simulink model "SWC_APP_type"  (R2024a)
settings: Solver=FixedStepDiscrete  StartTime=0.0  StopTime=10.0  FixedStep=0.001  RelTol=1e-3
values from neighbouring files (symbols this model uses):
  TRUE = boolean( 1 )    [vcu_local_hdr.m]
undefined symbols (not defined in the file or in its folder): KAPP_ADCKL15_enum, KAPP_ADCKL30_enum, KFOC_ADCFlyBackTemp_enum, KFOC_ADCMCUTemp_enum, KFOC_ADCMotorUTemp_enum, KFOC_ADCMotorVTemp_enum, KFOC_ADCMotorWTemp_enum, KFOC_ADCOilTemp_enum, KFOC_ADCSicUTemp_enum, KFOC_ADCSicVTemp_enum, KFOC_ADCSicWTemp_enum, KOPM_FakeKL15_flg
libraries: FVT_lib x19, crm_grc x1, eop_grc x1, halin x1, halout x1, inp x1, llc_grc x1, opm_grc x1, syl_grc x1, dgl_grc x1
(part 1 of 2)
settings Model: DataDictionary=APPTypes.sldd  Creator=FVT22063  LastModifiedBy=FVT24180
settings DataIOCC: SaveFormat=StructureWithTime
settings OptimizationCC: DefaultParameterBehavior=Inlined  EnhancedBackFolding=on  PassReuseOutputArgsAs=Individual arguments  ZeroExternalMemoryAtStartup=off  ZeroInternalMemoryAtStartup=off  OptimizeBlockOrder=speed  DifferentSizesBufferReuse=on  OptimizationCustomize=off  EfficientTunableParamExpr=on
settings DebuggingCC: ParameterTunabilityLossMsg=error
settings HardwareCC: ProdBitPerPointer=32  ProdBitPerSizeT=32  ProdBitPerPtrDiffT=32  ProdLargestAtomicInteger=Long  ProdLargestAtomicFloat=Double  ProdWordSize=32  ProdLongLongMode=on  ProdHWDeviceType=ARM Compatible->ARM Cortex-M
settings ModelReferenceCC: ModelReferenceNumInstancesAllowed=Single
settings SFSimCC: SimCustomHeaderCode="#include \"FVTMC_API.h\""  SimUserSources=FVTMC_API.c  MATLABDynamicMemAlloc=off
settings RTWCC: Description=AUTOSAR  SystemTargetFile=autosar.tlc  GenCodeOnly=on  TemplateMakefile=ert_default_tmf  PortableWordSizes=on
settings CodeAppCC: ForceParamTrailComments=on  IgnoreCustomStorageClasses=off  OperatorAnnotations=on  SimulinkDataObjDesc=on  SFDataObjDesc=on  InsertBlockDesc=on
settings STFCustomTargetCC: UtilityFuncGeneration=Shared location  MultiwordLength=256  ParMdlRefBuildCompliant=on  CompOptLevelCompliant=on  IncludeMdlTerminateFcn=off  CombineOutputUpdateFcns=on  SuppressErrorStatus=on  ERTCustomFileBanners=on  SupportNonFinite=off  SupportComplex=off  SupportContinuousTime=off  SupportNonInlinedSFcns=off  RemoveResetFunc=on  MATLABClassNameForMDSCustomization=Simulink.SoftwareTarget.ERTCustomization  AutosarCompliant=on  GRTInterface=off  GenerateSharedConstants=off  LookupTableObjectStructAxisOrder=2,1,3,4,...  LUTObjectStructOrderEvenSpacing=Size,Table,Breakpoints  SystemTargetFile=autosar.tlc
settings ERTTargetCC: TargetLangStandard=C99 (ISO)  UtilityFuncGeneration=Shared location  ConcurrentExecutionCompliant=off  IncludeMdlTerminateFcn=off  SuppressErrorStatus=on  SupportNonFinite=off  SupportComplex=off  ModelStepFunctionPrototypeControlCompliant=off  CPPClassGenCompliant=off  AutosarCompliant=on  GenerateSharedConstants=off  LookupTableObjectStructAxisOrder=2,1,3,4,...  LUTObjectStructOrderEvenSpacing=Size,Table,Breakpoints  GenerateASAP2=on  InlinedParameterPlacement=NonHierarchical  ERTCustomFileTemplate=example_file_process.tlc  ConvertIfToSwitch=off  SuppressUnreachableDefaultCases=off  BooleanTrueId=true_MatlabRTW  BooleanFalseId=false_MatlabRTW

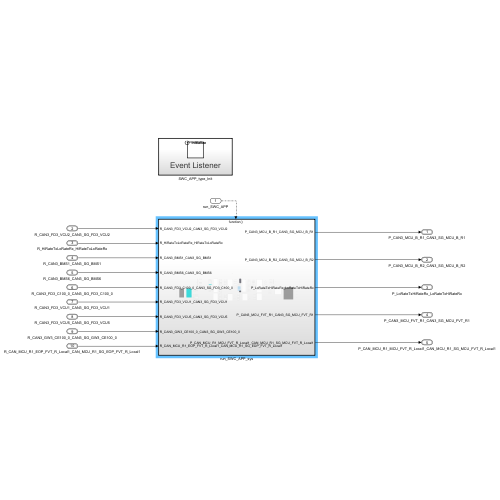
[thumbnail: Simulink's stored preview of the top-level diagram]
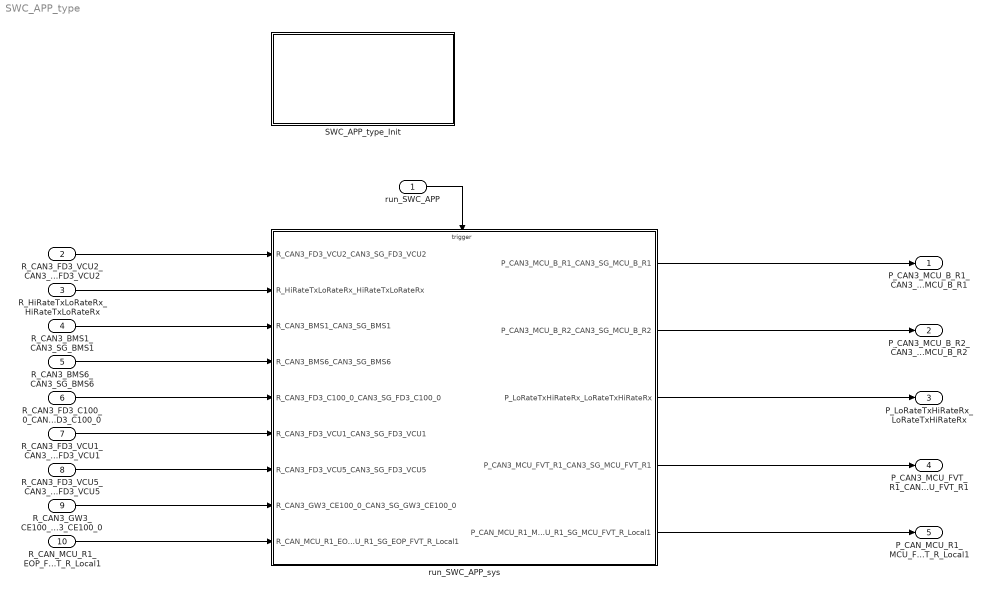
== system SWC_APP_type ==
  run_SWC_APP : Inport  SampleTime=0.001  OutputFunctionCall=on
  R_CAN3_FD3_VCU2_CAN3_SG_FD3_VCU2 : Inport  Port=2  OutDataTypeStr=Bus: DT_CAN3_SG_FD3_VCU2  PortDimensions=1  BusOutputAsStruct=on
  R_HiRateTxLoRateRx_HiRateTxLoRateRx : Inport  Port=3  OutDataTypeStr=Bus: DT_HiRateTxLoRateRx  PortDimensions=1  BusOutputAsStruct=on
  R_CAN3_BMS1_CAN3_SG_BMS1 : Inport  Port=4  OutDataTypeStr=Bus: DT_CAN3_SG_BMS1  PortDimensions=1  BusOutputAsStruct=on
  R_CAN3_BMS6_CAN3_SG_BMS6 : Inport  Port=5  OutDataTypeStr=Bus: DT_CAN3_SG_BMS6  PortDimensions=1  BusOutputAsStruct=on
  R_CAN3_FD3_C100_0_CAN3_SG_FD3_C100_0 : Inport  Port=6  OutDataTypeStr=Bus: DT_CAN3_SG_FD3_C100_0  PortDimensions=1  BusOutputAsStruct=on
  R_CAN3_FD3_VCU1_CAN3_SG_FD3_VCU1 : Inport  Port=7  OutDataTypeStr=Bus: DT_CAN3_SG_FD3_VCU1  PortDimensions=1  BusOutputAsStruct=on
  R_CAN3_FD3_VCU5_CAN3_SG_FD3_VCU5 : Inport  Port=8  OutDataTypeStr=Bus: DT_CAN3_SG_FD3_VCU5  PortDimensions=1  BusOutputAsStruct=on
  R_CAN3_GW3_CE100_0_CAN3_SG_GW3_CE100_0 : Inport  Port=9  OutDataTypeStr=Bus: DT_CAN3_SG_GW3_CE100_0  PortDimensions=1  BusOutputAsStruct=on
  R_CAN_MCU_R1_EOP_FVT_R_Local1_CAN_MCU_R1_SG_EOP_FVT_R_Local1 : Inport  Port=10  OutDataTypeStr=Bus: DT_CAN_MCU_R1_SG_EOP_FVT_R_Local1  PortDimensions=1  BusOutputAsStruct=on
  SWC_APP_type_Init : Subsystem
  run_SWC_APP_sys : Subsystem
  P_CAN3_MCU_B_R1_CAN3_SG_MCU_B_R1 : Outport  OutDataTypeStr=Bus: DT_CAN3_SG_MCU_B_R1  PortDimensions=1  BusOutputAsStruct=on
  P_CAN3_MCU_B_R2_CAN3_SG_MCU_B_R2 : Outport  Port=2  OutDataTypeStr=Bus: DT_CAN3_SG_MCU_B_R2  PortDimensions=1  BusOutputAsStruct=on
  P_LoRateTxHiRateRx_LoRateTxHiRateRx : Outport  Port=3  OutDataTypeStr=Bus: DT_LoRateTxHiRateRx  PortDimensions=1  BusOutputAsStruct=on
  P_CAN3_MCU_FVT_R1_CAN3_SG_MCU_FVT_R1 : Outport  Port=4  OutDataTypeStr=Bus: DT_CAN3_SG_MCU_FVT_R1  PortDimensions=1  BusOutputAsStruct=on
  P_CAN_MCU_R1_MCU_FVT_R_Local1_CAN_MCU_R1_SG_MCU_FVT_R_Local1 : Outport  Port=5  OutDataTypeStr=Bus: DT_CAN_MCU_R1_SG_MCU_FVT_R_Local1  PortDimensions=1  BusOutputAsStruct=on
  wires:
  R_CAN3_FD3_VCU2_CAN3_SG_FD3_VCU2/1 -> run_SWC_APP_sys/1(R_CAN3_FD3_VCU2_CAN3_SG_FD3_VCU2)
  R_HiRateTxLoRateRx_HiRateTxLoRateRx/1 -> run_SWC_APP_sys/2(R_HiRateTxLoRateRx_HiRateTxLoRateRx)
  run_SWC_APP_sys/1(P_CAN3_MCU_B_R1_CAN3_SG_MCU_B_R1) -> P_CAN3_MCU_B_R1_CAN3_SG_MCU_B_R1/1
  run_SWC_APP_sys/2(P_CAN3_MCU_B_R2_CAN3_SG_MCU_B_R2) -> P_CAN3_MCU_B_R2_CAN3_SG_MCU_B_R2/1
  run_SWC_APP_sys/3(P_LoRateTxHiRateRx_LoRateTxHiRateRx) -> P_LoRateTxHiRateRx_LoRateTxHiRateRx/1
  run_SWC_APP/1 -> run_SWC_APP_sys/Trigger
  R_CAN3_BMS1_CAN3_SG_BMS1/1 -> run_SWC_APP_sys/3(R_CAN3_BMS1_CAN3_SG_BMS1)
  R_CAN3_BMS6_CAN3_SG_BMS6/1 -> run_SWC_APP_sys/4(R_CAN3_BMS6_CAN3_SG_BMS6)
  R_CAN3_FD3_C100_0_CAN3_SG_FD3_C100_0/1 -> run_SWC_APP_sys/5(R_CAN3_FD3_C100_0_CAN3_SG_FD3_C100_0)
  R_CAN3_FD3_VCU1_CAN3_SG_FD3_VCU1/1 -> run_SWC_APP_sys/6(R_CAN3_FD3_VCU1_CAN3_SG_FD3_VCU1)
  R_CAN3_FD3_VCU5_CAN3_SG_FD3_VCU5/1 -> run_SWC_APP_sys/7(R_CAN3_FD3_VCU5_CAN3_SG_FD3_VCU5)
  R_CAN3_GW3_CE100_0_CAN3_SG_GW3_CE100_0/1 -> run_SWC_APP_sys/8(R_CAN3_GW3_CE100_0_CAN3_SG_GW3_CE100_0)
  run_SWC_APP_sys/4(P_CAN3_MCU_FVT_R1_CAN3_SG_MCU_FVT_R1) -> P_CAN3_MCU_FVT_R1_CAN3_SG_MCU_FVT_R1/1
  R_CAN_MCU_R1_EOP_FVT_R_Local1_CAN_MCU_R1_SG_EOP_FVT_R_Local1/1 -> run_SWC_APP_sys/9(R_CAN_MCU_R1_EOP_FVT_R_Local1_CAN_MCU_R1_SG_EOP_FVT_R_Local1)
  run_SWC_APP_sys/5(P_CAN_MCU_R1_MCU_FVT_R_Local1_CAN_MCU_R1_SG_MCU_FVT_R_Local1) -> P_CAN_MCU_R1_MCU_FVT_R_Local1_CAN_MCU_R1_SG_MCU_FVT_R_Local1/1

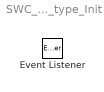
== system SWC_APP_type/SWC_APP_type_Init ==
  Event Listener : EventListener  EventName=reset

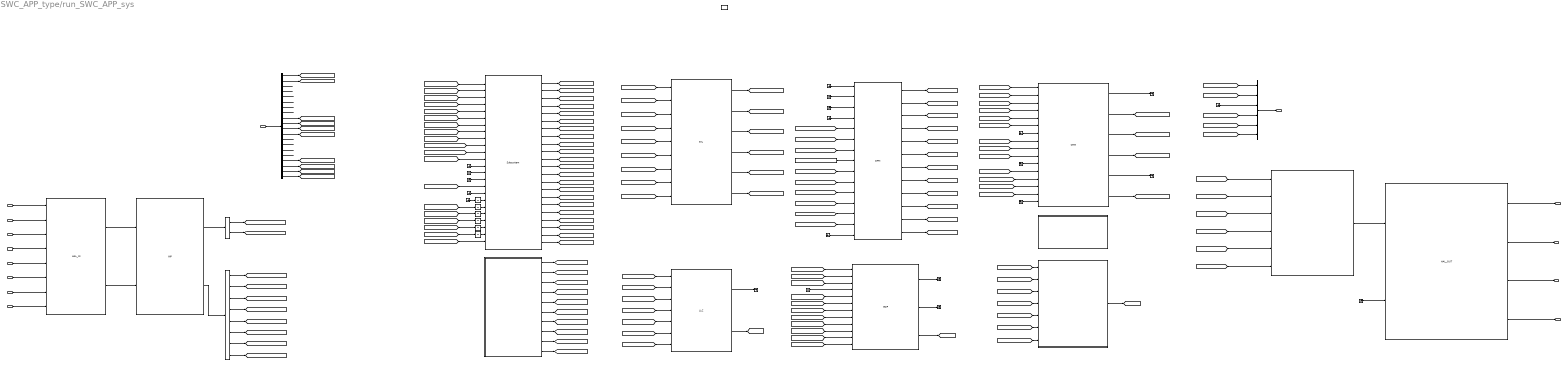
== system SWC_APP_type/run_SWC_APP_sys ==
  note: No use
  note: No use
  R_CAN3_FD3_VCU2_CAN3_SG_FD3_VCU2 : Inport
  R_HiRateTxLoRateRx_HiRateTxLoRateRx : Inport  Port=2
  R_CAN3_BMS1_CAN3_SG_BMS1 : Inport  Port=3
  R_CAN3_BMS6_CAN3_SG_BMS6 : Inport  Port=4
  R_CAN3_FD3_C100_0_CAN3_SG_FD3_C100_0 : Inport  Port=5
  R_CAN3_FD3_VCU1_CAN3_SG_FD3_VCU1 : Inport  Port=6
  R_CAN3_FD3_VCU5_CAN3_SG_FD3_VCU5 : Inport  Port=7
  R_CAN3_GW3_CE100_0_CAN3_SG_GW3_CE100_0 : Inport  Port=8
  R_CAN_MCU_R1_EOP_FVT_R_Local1_CAN_MCU_R1_SG_EOP_FVT_R_Local1 : Inport  Port=9
  function : TriggerPort  TriggerType=function-call  VariantControl=(inherit)  SampleTimeType=periodic  SampleTime=-1
  Bus Creator : BusCreator  Inputs=6  OutDataTypeStr=Bus: DT_LoRateTxHiRateRx  NonVirtualBus=on
  Bus Selector : BusSelector  OutputSignals=f32_DSS_uDCSide,f32_RotS_nRot,f32_RotS_agRot,f32_PCS_iPaCS,f32_PCS_iPbCS,f32_PCS_iPcCS,u8_PCS_bOverCurr,f32_TorqEst_tqMotEst,f32_CCM_uDVoltTar,f32_CCM_uQVoltTar,f32_CCM_iDCurrAct,f32_CCM_iQCurrAct,u8_Diag_bPhaCurrOverU,u8_Diag_bPhaCurrOverV,u8_Diag_bPhaCurrOverW,u8_Diag1_b1_SumErr_null,f32_VCCM_BattVolCirRadius_V,f32_VCCM_VcmdBfLim_V,f32_VMCM_TqAct_Nm,u8_VDSM_FltActn12_flg
  Bus Selector1 : BusSelector  OutputSignals=VINP_ActiveDischReq_flg,VINP_HVBContactorSta_flg,VINP_FDCVCURrTMCtrlModeReq_enum,VINP_RrMCUEnaReq_flg,VINP_ShiftGearPosn_enum,VINP_RrActvDmpDisabReq_flg,VINP_RrCoolanttemp_C,VINP_RrCoolantflow_Lpmin
  Bus Selector2 : BusSelector  OutputSignals=VINP_EOPFVTRActualSpdSta_rpm,VINP_EOPFVTRRunStatusSta_enum
  CRM : crm_grc/CRM  SystemSampleTime=-1  VariantActivationTime=update diagram  AllowFlexibleInterface=on  Latency=0  AutoFrameSizeCalculation=off
  Constant3 : Constant  Value=KOPM_FakeKL15_flg
  EOP : eop_grc/EOP  SystemSampleTime=-1  VariantActivationTime=update diagram  AllowFlexibleInterface=on  Latency=0  AutoFrameSizeCalculation=off
  GateDirver_Temp_Read : Subsystem  TreatAsAtomicUnit=on
      settings: RTWSystemCode=Nonreusable function  RTWFcnNameOpts=Use subsystem name  RTWFileNameOpts=Use subsystem name
  Ground{,1..10,17..21} (16 alike) : Ground
  HAL_IN : halin/HAL_IN  SystemSampleTime=-1  VariantActivationTime=update diagram  AllowFlexibleInterface=on  Latency=0  AutoFrameSizeCalculation=off
  HAL_OUT : halout/HAL_OUT  SystemSampleTime=-1  VariantActivationTime=update diagram  AllowFlexibleInterface=on  Latency=0  AutoFrameSizeCalculation=off
  INP : inp/INP  SystemSampleTime=-1  VariantActivationTime=update diagram  AllowFlexibleInterface=on  Latency=0  AutoFrameSizeCalculation=off
  LLC : llc_grc/LLC  SystemSampleTime=-1  VariantActivationTime=update diagram  AllowFlexibleInterface=on  Latency=0  AutoFrameSizeCalculation=off
  OPM : opm_grc/OPM  SystemSampleTime=-1  VariantActivationTime=update diagram  AllowFlexibleInterface=on  Latency=0  AutoFrameSizeCalculation=off
  OUTP : Subsystem
  SYL : syl_grc/SYL  SystemSampleTime=-1  VariantActivationTime=update diagram  AllowFlexibleInterface=on  Latency=0  AutoFrameSizeCalculation=off
  Subsystem : dgl_grc/Subsystem  SystemSampleTime=-1  VariantActivationTime=update diagram  AllowFlexibleInterface=on  Latency=0  AutoFrameSizeCalculation=off
  Subsystem1 : Subsystem
  Subsystem2 : Subsystem
  Terminator{,2..5} (5 alike) : Terminator
  Unit Delay{,1..5} (6 alike) : UnitDelay  SampleTime=-1  HasFrameUpgradeWarning=on
  P_CAN3_MCU_B_R1_CAN3_SG_MCU_B_R1 : Outport
  P_CAN3_MCU_B_R2_CAN3_SG_MCU_B_R2 : Outport  Port=2
  P_LoRateTxHiRateRx_LoRateTxHiRateRx : Outport  Port=3
  P_CAN3_MCU_FVT_R1_CAN3_SG_MCU_FVT_R1 : Outport  Port=4
  P_CAN_MCU_R1_MCU_FVT_R_Local1_CAN_MCU_R1_SG_MCU_FVT_R_Local1 : Outport  Port=5
  wires:
  R_CAN3_FD3_VCU2_CAN3_SG_FD3_VCU2/1 -> HAL_IN/6
  R_HiRateTxLoRateRx_HiRateTxLoRateRx/1 -> Bus Selector/1
  Bus Selector/1 -> [DSS_uDCSide]  "<f32_DSS_uDCSide>"
  Bus Selector/2 -> [RotS_nRot]  "<f32_RotS_nRot>"
  Bus Selector/3 -> ?  "<f32_RotS_agRot>"
  Bus Selector/4 -> ?  "<f32_PCS_iPaCS>"
  Bus Selector/5 -> ?  "<f32_PCS_iPbCS>"
  Bus Selector/6 -> ?  "<f32_PCS_iPcCS>"
  Bus Selector/7 -> ?  "<u8_PCS_bOverCurr>"
  Bus Selector/8 -> ?  "<f32_TorqEst_tqMotEst>"
  Bus Selector/9 -> [uDVoltTar]  "<f32_CCM_uDVoltTar>"
  Bus Selector/10 -> [uQVoltTar]  "<f32_CCM_uQVoltTar>"
  Bus Selector/11 -> [iDCurrAct]  "<f32_CCM_iDCurrAct>"
  Bus Selector/12 -> [iQCurrAct]  "<f32_CCM_iQCurrAct>"
  Bus Selector/13 -> ?  "<u8_Diag_bPhaCurrOverU>"
  Bus Selector/14 -> ?  "<u8_Diag_bPhaCurrOverV>"
  Bus Selector/15 -> ?  "<u8_Diag_bPhaCurrOverW>"
  Bus Selector/16 -> ?  "<u8_Diag1_b1_SumErr_null>"
  Bus Selector/17 -> [VCCM_BattVolCirRadius_V]  "<f32_VCCM_BattVolCirRadius_V>"
  Bus Selector/18 -> [VCCM_VcmdBfLim_V]  "<f32_VCCM_VcmdBfLim_V>"
  Bus Selector/19 -> [VMCM_TqAct_Nm]  "<f32_VMCM_TqAct_Nm>"
  Bus Selector/20 -> [VDSM_FltActn12_flg]  "<u8_VDSM_FltActn12_flg>"
  Ground/1 -> Bus Creator/3
  [RotS_nRot] -> OPM/5
  [DSS_uDCSide] -> OPM/6
  Ground1/1 -> OPM/1
  Ground2/1 -> OPM/2
  Ground4/1 -> OPM/4
  Ground3/1 -> OPM/3
  Ground5/1 -> OPM/15
  Bus Creator/1 -> P_LoRateTxHiRateRx_LoRateTxHiRateRx/1
  OPM/7 -> [OpMod_bTMReady]  "OpMod_bTMReady"
  OPM/2 -> [OpMod_stMotAct]  "OpMod_stMotAct"
  OPM/6 -> [OpMod_bDchaCmpl]  "OpMod_bDchaCmpl"
  OPM/1 -> [OpMod_stIvtrTar]  "OpMod_stIvtrTar"
  OPM/3 -> [OpMod_stTMOper]  "OpMod_stTMOper"
  OPM/4 -> [OpMod_bMCUEna]  "OpMod_bMCUEna"
  OPM/5 -> [OpMod_bReadyPreDcha]  "OpMod_bReadyPreDcha"
  OPM/8 -> [OpMod_bPasDchaEna]  "Opmod_bPsvDischrgEna"
  OPM/11 -> [CurLoopEna]
  OPM/10 -> [OpMod_bBoostOPSta]  "OpMod_bBoostOPSta"
  OPM/9 -> [OpMod_bHeatingOPSta]  "OpMod_bHeatingOPSta"
  [OpMod_stMotAct] -> Bus Creator/1
  [OpMod_stIvtrTar] -> Bus Creator/2
  Subsystem/1 -> [OverSpdCoef]
  Subsystem/2 -> [IGBTCoef]
  Subsystem/16 -> [Diag3_b1_TempOilFault_null]
  Subsystem/17 -> [Diag2_b1_HVOverErr_null]
  Subsystem/18 -> [Diag2_b1_HVLowErr_null]
  Subsystem/19 -> [DiagM_bOverTorque]
  Subsystem/20 -> [DiagM_bEOPFlt]
  Subsystem/21 -> [DiagM_bOver2Stop]
  Subsystem/22 -> [DiagM_bZeroCurr]
  Subsystem/3 -> [MotCoef]
  Subsystem/4 -> [PCBCoef]
  Subsystem/5 -> [OilCoef]
  Subsystem/6 -> [UdcOverCoef]
  Subsystem/7 -> [UdcLowCoef]
  Subsystem/8 -> [DiagM_Fault2Level]
  Subsystem/9 -> [DiagM_bStallProt]
  Subsystem/10 -> [DiagM_b1_OverSpdErr_null]
  Subsystem/11 -> [Diag3_b1_TempMotWarning_null]
  Subsystem/12 -> [Diag3_b1_TempMotFault_null]
  Subsystem/13 -> [Diag3_b1_TempIGBTFault_null]
  Subsystem/14 -> [Diag3_b1_TempIGBTWarning_null]
  Subsystem/15 -> [Diag3_b1_TempPCBFault_null]
  [RotS_nRot] -> Subsystem/1
  [DSS_uDCSide] -> Subsystem/2
  [CurLoopEna] -> Unit Delay/1
  [VCU_bActvDmpDiReq] -> Subsystem/24
  [VFOC_ADCMCUTemp_degC] -> Subsystem/3
  [VFOC_ADCSicUTemp_degC] -> Subsystem/4
  [VFOC_ADCSicVTemp_degC] -> Subsystem/5
  [VINP_FDCVCURrTMCtrlModeReq_enum] -> Subsystem/10
  Ground20/1 -> Unit Delay5/1
  [VMCM_IqCmd_A] -> Unit Delay1/1
  [VFOC_ADCSicWTemp_degC] -> Subsystem/6
  [VFOC_ADCMotorWTemp_degC] -> Subsystem/9
  [VDSM_FltActn12_flg] -> Subsystem/16
  [SysLim_tqTMTqMax] -> Unit Delay4/1
  [VINP_HVBContactorSta_flg] -> Subsystem/11
  [VFOC_ADCMotorVTemp_degC] -> Subsystem/8
  Ground21/1 -> Subsystem/17
  Ground17/1 -> Subsystem/13
  Ground18/1 -> Subsystem/14
  [SysLim_tqTMTqMin] -> Unit Delay3/1
  [VMCM_IdCmd_A] -> Unit Delay2/1
  [VFOC_ADCOilTemp_degC] -> Subsystem/12
  Ground19/1 -> Subsystem/15
  [VFOC_ADCMotorUTemp_degC] -> Subsystem/7
  SYL/1 -> [SysLim_tqTMTqMax]
  SYL/2 -> [SysLim_tqTMTqMin]
  SYL/3 -> [SysLim_nTMSpdMin]
  SYL/4 -> [SysLim_nTMSpdMax]
  SYL/5 -> [SysLim_frqSwitchMax]
  [RotS_nRot] -> SYL/1
  [DSS_uDCSide] -> SYL/2
  [OverSpdCoef] -> SYL/3
  [IGBTCoef] -> SYL/4
  [MotCoef] -> SYL/5
  [PCBCoef] -> SYL/6
  [OilCoef] -> SYL/7
  [UdcOverCoef] -> SYL/8
  [UdcLowCoef] -> SYL/9
  Unit Delay/1 -> Subsystem/23
  Unit Delay1/1 -> Subsystem/22
  Unit Delay2/1 -> Subsystem/21
  Unit Delay3/1 -> Subsystem/20
  Unit Delay4/1 -> Subsystem/19
  Unit Delay5/1 -> Subsystem/18
  CRM/3 -> [VMCM_IdCmd_A]
  CRM/4 -> [VMCM_IqCmd_A]
  [VMCM_IdCmd_A] -> Bus Creator/4
  [VMCM_IqCmd_A] -> Bus Creator/5
  [DiagM_Fault2Level] -> Bus Creator/6
  CRM/1 -> Terminator/1
  CRM/2 -> [CurrM_pwrTMPwrEst]
  CRM/5 -> Terminator2/1
  [iQCurrAct] -> CRM/4
  [uQVoltTar] -> CRM/2
  [iDCurrAct] -> CRM/3
  [uDVoltTar] -> CRM/1
  [DSS_uDCSide] -> CRM/5
  [RotS_nRot] -> CRM/6
  [CurLoopEna] -> CRM/8
  [VCCM_VcmdBfLim_V] -> CRM/10
  [VCCM_BattVolCirRadius_V] -> CRM/9
  Ground6/1 -> CRM/11
  Ground7/1 -> CRM/7
  [OpMod_stMotAct] -> CRM/12
  [SysLim_tqTMTqMax] -> CRM/13
  [SysLim_tqTMTqMin] -> CRM/14
  [DiagM_bZeroCurr] -> CRM/15
  Ground8/1 -> CRM/16
  [DiagM_bOver2Stop] -> OPM/7
  Constant3/1 -> OPM/8
  [VINP_ShiftGearPosn_enum] -> OPM/10
  [VINP_RrMCUEnaReq_flg] -> OPM/12
  [VINP_RrActvDmpDisabReq_flg] -> OPM/11
  [VINP_ActiveDischReq_flg] -> OPM/9
  Subsystem1/1(VFOC_ADCMCUTemp_degC) -> [VFOC_ADCMCUTemp_degC]
  Subsystem1/2(VFOC_ADCOilTemp_degC) -> [VFOC_ADCOilTemp_degC]
  Subsystem1/3(VFOC_ADCMotorUTemp_degC) -> [VFOC_ADCMotorUTemp_degC]
  Subsystem1/4(VFOC_ADCMotorVTemp_degC) -> [VFOC_ADCMotorVTemp_degC]
  Subsystem1/5(VFOC_ADCMotorWTemp_degC) -> [VFOC_ADCMotorWTemp_degC]
  Subsystem1/6(VFOC_ADCSicUTemp_degC) -> [VFOC_ADCSicUTemp_degC]
  Subsystem1/7(VFOC_ADCSicVTemp_degC) -> [VFOC_ADCSicVTemp_degC]
  Subsystem1/8(VFOC_ADCSicWTemp_degC) -> [VFOC_ADCSicWTemp_degC]
  R_CAN3_BMS1_CAN3_SG_BMS1/1 -> HAL_IN/2
  R_CAN3_FD3_VCU5_CAN3_SG_FD3_VCU5/1 -> HAL_IN/7
  [iDCurrAct] -> Subsystem2/1(iDCurrAct)
  [iQCurrAct] -> Subsystem2/2(iQCurrAct)
  Subsystem1/9(ADCKL30) -> [ADCKL30]
  Subsystem1/10(ADCKL15) -> [ADCKL15]
  [ADCKL30] -> Subsystem2/3(ADCKL30)
  [ADCKL15] -> Subsystem2/4(ADCKL15)
  [DSS_uDCSide] -> Subsystem2/5(DSS_uDCSide)
  [VFOC_ADCOilTemp_degC] -> Subsystem2/7(OilTemp)
  [RotS_nRot] -> Subsystem2/6(RotS_nRot)
  Subsystem2/1(BAPP_outputs) -> [BAPP_outputs]
  OPM/12 -> [BOPM_outputs]
  SYL/6 -> [BSYL_outputs]
  CRM/6 -> [BCRM_outputs]
  EOP/3 -> [BEOP_outputs]
  EOP/2 -> Terminator3/1
  EOP/1 -> Terminator4/1
  LLC/1 -> Terminator5/1
  LLC/2 -> [BLLC_outputs]
  [VFOC_ADCSicUTemp_degC] -> EOP/1
  [VFOC_ADCSicVTemp_degC] -> EOP/2
  [VFOC_ADCSicWTemp_degC] -> EOP/3
  [VFOC_ADCMotorVTemp_degC] -> EOP/5
  [VFOC_ADCMotorWTemp_degC] -> EOP/6
  Ground9/1 -> EOP/4
  [VFOC_ADCOilTemp_degC] -> EOP/7
  [VFOC_ADCSicUTemp_degC] -> LLC/1
  [VFOC_ADCSicVTemp_degC] -> LLC/2
  [VFOC_ADCSicWTemp_degC] -> LLC/3
  [VFOC_ADCOilTemp_degC] -> LLC/6
  [CurrM_pwrTMPwrEst] -> LLC/7
  [BAPP_outputs] -> OUTP/1(BAPP_outputs)
  [BCRM_outputs] -> OUTP/2(BCRM_outputs)
  [BEOP_outputs] -> OUTP/3(BEOP_outputs)
  [BLLC_outputs] -> OUTP/4(BLLC_outputs)
  [BOPM_outputs] -> OUTP/5(BOPM_outputs)
  [BSYL_outputs] -> OUTP/6(BSYL_outputs)
  OUTP/1(BOUTP_outputs) -> HAL_OUT/1
  HAL_OUT/1 -> P_CAN3_MCU_B_R1_CAN3_SG_MCU_B_R1/1
  HAL_OUT/2 -> P_CAN3_MCU_B_R2_CAN3_SG_MCU_B_R2/1
  HAL_OUT/3 -> P_CAN3_MCU_FVT_R1_CAN3_SG_MCU_FVT_R1/1
  HAL_OUT/4 -> P_CAN_MCU_R1_MCU_FVT_R_Local1_CAN_MCU_R1_SG_MCU_FVT_R_Local1/1
  Ground10/1 -> HAL_OUT/2
  R_CAN_MCU_R1_EOP_FVT_R_Local1_CAN_MCU_R1_SG_EOP_FVT_R_Local1/1 -> HAL_IN/1
  R_CAN3_BMS6_CAN3_SG_BMS6/1 -> HAL_IN/3
  R_CAN3_FD3_C100_0_CAN3_SG_FD3_C100_0/1 -> HAL_IN/4
  R_CAN3_FD3_VCU1_CAN3_SG_FD3_VCU1/1 -> HAL_IN/5
  R_CAN3_GW3_CE100_0_CAN3_SG_GW3_CE100_0/1 -> HAL_IN/8
  HAL_IN/1 -> INP/1
  HAL_IN/2 -> INP/2
  INP/2 -> Bus Selector1/1
  Bus Selector1/1 -> [VINP_ActiveDischReq_flg]  "<VINP_ActiveDischReq_flg>"
  Bus Selector1/5 -> [VINP_ShiftGearPosn_enum]  "<VINP_ShiftGearPosn_enum>"
  Bus Selector1/2 -> [VINP_HVBContactorSta_flg]  "<VINP_HVBContactorSta_flg>"
  Bus Selector1/3 -> [VINP_FDCVCURrTMCtrlModeReq_enum]  "<VINP_FDCVCURrTMCtrlModeReq_enum>"
  Bus Selector1/4 -> [VINP_RrMCUEnaReq_flg]  "<VINP_RrMCUEnaReq_flg>"
  [VINP_HVBContactorSta_flg] -> OPM/14
  [VINP_FDCVCURrTMCtrlModeReq_enum] -> OPM/13
  Bus Selector1/6 -> [VINP_RrActvDmpDisabReq_flg]  "<VINP_RrActvDmpDisabReq_flg>"
  Bus Selector1/8 -> [VINP_RrCoolantflow_Lpmin]  "<VINP_RrCoolantflow_Lpmin>"
  Bus Selector1/7 -> [VINP_RrCoolanttemp_C]  "<VINP_RrCoolanttemp_C>"
  [VINP_RrCoolantflow_Lpmin] -> LLC/5
  [VINP_RrCoolanttemp_C] -> LLC/4
  [VINP_RrCoolanttemp_C] -> EOP/8
  INP/1 -> Bus Selector2/1
  [VMCM_TqAct_Nm] -> EOP/11
  [RotS_nRot] -> EOP/12
  Bus Selector2/1 -> [VINP_EOPFVTRActualSpdSta_rpm]  "<VINP_EOPFVTRActualSpdSta_rpm>"
  Bus Selector2/2 -> [VINP_EOPFVTRRunStatusSta_enum]  "<VINP_EOPFVTRRunStatusSta_enum>"
  [VINP_EOPFVTRRunStatusSta_enum] -> EOP/10
  [VINP_EOPFVTRActualSpdSta_rpm] -> EOP/9

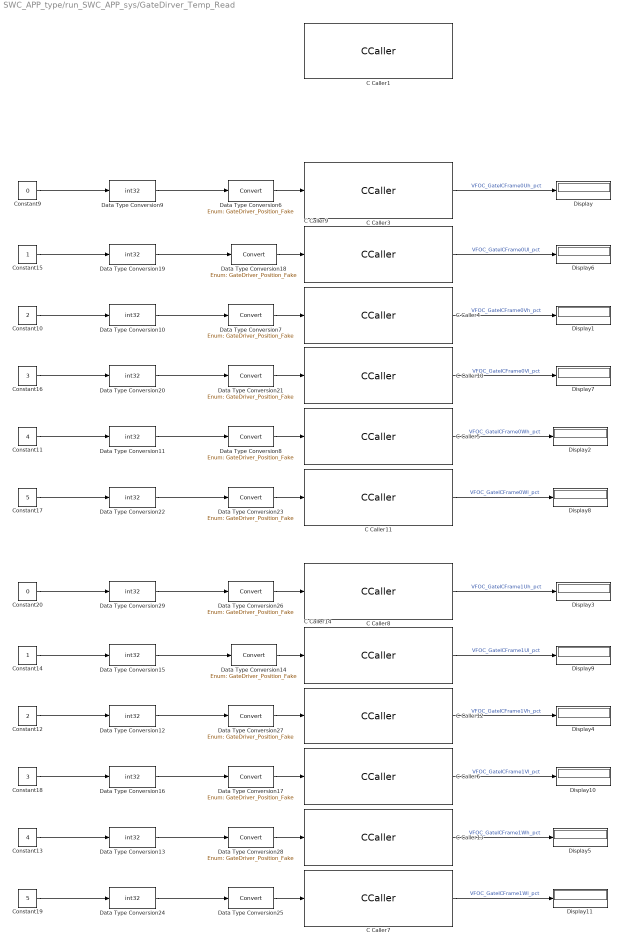
== system SWC_APP_type/run_SWC_APP_sys/GateDirver_Temp_Read ==
  C Caller1 : CCaller  FunctionName=update_gatedriver_data_duty
  C Caller{3..5,9..11} (6 alike) : CCaller  FunctionName=get_gatedriver_data_diagnostic1  PortSpecificationStruct="%)30     .    X ,   8    (     @         %    \"     (    !     0         %  0 \"0    $    _    07)G3F%M90  4&]R=$YA;64 4V-O<&4     26YD97@     5'EP90      4VEZ90      27-';&]B86P   X    P    !@    @    $          4    (     0    ,    !         !   P!O=70 #@   #     &    \"     0         !0    @    !     P    $         $  # &]U=  .    .     8    (    !          %    \"     $    &     0         0    !@   $]U='!U=   #@   #@    &    \"     8         !0    @    !     0    $         \"0    @               X    X    !@    @    $          4    (     0    8    !         !     &    <VEN9VQE   .    ,     8    (    !          %    \"     $    !     0         0  $ ,0    X    P    !@    @    ) @        4    (     0    $    !          (  0      #@   #@    &    \"     0         !0    @    !    \"     $         $     @   !P;W-I=&EO;@X    X    !@    @    $          4    (     0    @    !         !     (    <&]S:71I;VX.    .     8    (    !          %    \"     $    %     0         0    !0   $EN<'5T    #@   #@    &    \"     8         !0    @    !     0    $         \"0    @               X   !0    !@    @    $          4    (     0   !X    !         !     >    16YU;3H@1V%T941R:79E<E]0;W-I=&EO;E]&86ME   .    ,     8    (    !          %    \"     $    !     0         0  $ ,0    X    P    !@    @    ) @        4    (     0    $    !          (  0"
  C Caller{6..8,12..14} (6 alike) : CCaller  FunctionName=get_gatedriver_data_diagnostic2  PortSpecificationStruct="%)30     .    X ,   8    (     @         %    \"     (    !     0         %  0 \"0    $    _    07)G3F%M90  4&]R=$YA;64 4V-O<&4     26YD97@     5'EP90      4VEZ90      27-';&]B86P   X    P    !@    @    $          4    (     0    ,    !         !   P!O=70 #@   #     &    \"     0         !0    @    !     P    $         $  # &]U=  .    .     8    (    !          %    \"     $    &     0         0    !@   $]U='!U=   #@   #@    &    \"     8         !0    @    !     0    $         \"0    @               X    X    !@    @    $          4    (     0    8    !         !     &    <VEN9VQE   .    ,     8    (    !          %    \"     $    !     0         0  $ ,0    X    P    !@    @    ) @        4    (     0    $    !          (  0      #@   #@    &    \"     0         !0    @    !    \"     $         $     @   !P;W-I=&EO;@X    X    !@    @    $          4    (     0    @    !         !     (    <&]S:71I;VX.    .     8    (    !          %    \"     $    %     0         0    !0   $EN<'5T    #@   #@    &    \"     8         !0    @    !     0    $         \"0    @               X   !0    !@    @    $          4    (     0   !X    !         !     >    16YU;3H@1V%T941R:79E<E]0;W-I=&EO;E]&86ME   .    ,     8    (    !          %    \"     $    !     0         0  $ ,0    X    P    !@    @    ) @        4    (     0    $    !          (  0"
  Constant10 : Constant  Value=2
  Constant11 : Constant  Value=4
  Constant12 : Constant  Value=2
  Constant13 : Constant  Value=4
  Constant14 : Constant
  Constant15 : Constant
  Constant16 : Constant  Value=3
  Constant17 : Constant  Value=5
  Constant18 : Constant  Value=3
  Constant19 : Constant  Value=5
  Constant20 : Constant  Value=0
  Constant9 : Constant  Value=0
  Data Type Conversion{9..13,15..16,19..20,22,24,29} (12 alike) : DataTypeConversion  OutDataTypeStr=int32  SaturateOnIntegerOverflow=off  RndMeth=Floor
  Data Type Conversion{6..8,14,17..18,21,23,26..28} (11 alike) : DataTypeConversion  OutDataTypeStr=Enum: GateDriver_Position_Fake  SaturateOnIntegerOverflow=off  RndMeth=Floor
  Data Type Conversion25 : DataTypeConversion  SaturateOnIntegerOverflow=off  RndMeth=Floor
  Display{,1..11} (12 alike) : Display
  wires:
  Data Type Conversion11/1 -> Data Type Conversion8/1
  Constant10/1 -> Data Type Conversion10/1
  Data Type Conversion8/1 -> C Caller5/1
  Data Type Conversion9/1 -> Data Type Conversion6/1
  Data Type Conversion10/1 -> Data Type Conversion7/1
  Data Type Conversion6/1 -> C Caller3/1
  Constant9/1 -> Data Type Conversion9/1
  Data Type Conversion7/1 -> C Caller4/1
  Constant11/1 -> Data Type Conversion11/1
  C Caller3/1 -> Display/1  "VFOC_GateICFrame0Uh_pct"
  C Caller4/1 -> Display1/1  "VFOC_GateICFrame0Vh_pct"
  C Caller5/1 -> Display2/1  "VFOC_GateICFrame0Wh_pct"
  C Caller9/1 -> Display6/1  "VFOC_GateICFrame0Ul_pct"
  Data Type Conversion18/1 -> C Caller9/1
  Constant15/1 -> Data Type Conversion19/1
  Data Type Conversion19/1 -> Data Type Conversion18/1
  Constant16/1 -> Data Type Conversion20/1
  C Caller10/1 -> Display7/1  "VFOC_GateICFrame0Vl_pct"
  Data Type Conversion21/1 -> C Caller10/1
  Data Type Conversion20/1 -> Data Type Conversion21/1
  C Caller11/1 -> Display8/1  "VFOC_GateICFrame0Wl_pct"
  Constant17/1 -> Data Type Conversion22/1
  Data Type Conversion23/1 -> C Caller11/1
  Data Type Conversion22/1 -> Data Type Conversion23/1
  C Caller14/1 -> Display9/1  "VFOC_GateICFrame1Ul_pct"
  Data Type Conversion24/1 -> Data Type Conversion25/1
  Data Type Conversion25/1 -> C Caller7/1
  C Caller13/1 -> Display5/1  "VFOC_GateICFrame1Wh_pct"
  C Caller6/1 -> Display10/1  "VFOC_GateICFrame1Vl_pct"
  Data Type Conversion16/1 -> Data Type Conversion17/1
  Data Type Conversion14/1 -> C Caller14/1
  C Caller12/1 -> Display4/1  "VFOC_GateICFrame1Vh_pct"
  Data Type Conversion26/1 -> C Caller8/1
  Constant12/1 -> Data Type Conversion12/1
  Data Type Conversion13/1 -> Data Type Conversion28/1
  Data Type Conversion27/1 -> C Caller12/1
  Constant19/1 -> Data Type Conversion24/1
  Constant14/1 -> Data Type Conversion15/1
  Constant13/1 -> Data Type Conversion13/1
  Constant18/1 -> Data Type Conversion16/1
  Data Type Conversion12/1 -> Data Type Conversion27/1
  Constant20/1 -> Data Type Conversion29/1
  Data Type Conversion29/1 -> Data Type Conversion26/1
  C Caller7/1 -> Display11/1  "VFOC_GateICFrame1Wl_pct"
  Data Type Conversion17/1 -> C Caller6/1
  Data Type Conversion28/1 -> C Caller13/1
  C Caller8/1 -> Display3/1  "VFOC_GateICFrame1Uh_pct"
  Data Type Conversion15/1 -> Data Type Conversion14/1

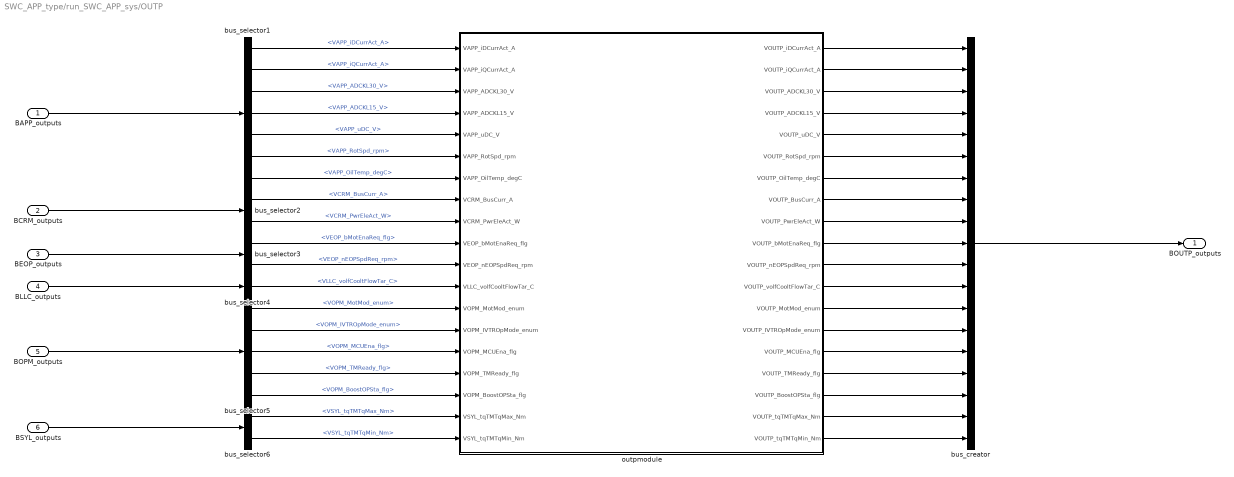
== system SWC_APP_type/run_SWC_APP_sys/OUTP ==
  BAPP_outputs : Inport  OutDataTypeStr=Bus: BAPP_outputs
  BCRM_outputs : Inport  Port=2  OutDataTypeStr=Bus: BCRM_outputs
  BEOP_outputs : Inport  Port=3  OutDataTypeStr=Bus: BEOP_outputs
  BLLC_outputs : Inport  Port=4  OutDataTypeStr=Bus: BLLC_outputs
  BOPM_outputs : Inport  Port=5  OutDataTypeStr=Bus: BOPM_outputs
  BSYL_outputs : Inport  Port=6  OutDataTypeStr=Bus: BSYL_outputs
  bus_creator : BusCreator  Inputs=19
  bus_selector1 : BusSelector  OutputSignals=VAPP_iDCurrAct_A,VAPP_iQCurrAct_A,VAPP_ADCKL30_V,VAPP_ADCKL15_V,VAPP_uDC_V,VAPP_RotSpd_rpm,VAPP_OilTemp_degC
  bus_selector2 : BusSelector  OutputSignals=VCRM_BusCurr_A,VCRM_PwrEleAct_W
  bus_selector3 : BusSelector  OutputSignals=VEOP_bMotEnaReq_flg,VEOP_nEOPSpdReq_rpm
  bus_selector4 : BusSelector  OutputSignals=VLLC_volfCooltFlowTar_C
  bus_selector5 : BusSelector  OutputSignals=VOPM_MotMod_enum,VOPM_IVTROpMode_enum,VOPM_MCUEna_flg,VOPM_TMReady_flg,VOPM_BoostOPSta_flg
  bus_selector6 : BusSelector  OutputSignals=VSYL_tqTMTqMax_Nm,VSYL_tqTMTqMin_Nm
  outpmodule : Subsystem
  BOUTP_outputs : Outport  OutDataTypeStr=Bus: BOUTP_outputs
  wires:
  outpmodule/16(VOUTP_TMReady_flg) -> bus_creator/16
  outpmodule/13(VOUTP_MotMod_enum) -> bus_creator/13
  outpmodule/15(VOUTP_MCUEna_flg) -> bus_creator/15
  outpmodule/14(VOUTP_IVTROpMode_enum) -> bus_creator/14
  bus_creator/1 -> BOUTP_outputs/1
  outpmodule/18(VOUTP_tqTMTqMax_Nm) -> bus_creator/18
  outpmodule/17(VOUTP_BoostOPSta_flg) -> bus_creator/17
  bus_selector5/2 -> outpmodule/14(VOPM_IVTROpMode_enum)  "<VOPM_IVTROpMode_enum>"
  bus_selector5/4 -> outpmodule/16(VOPM_TMReady_flg)  "<VOPM_TMReady_flg>"
  bus_selector4/1 -> outpmodule/12(VLLC_volfCooltFlowTar_C)  "<VLLC_volfCooltFlowTar_C>"
  BEOP_outputs/1 -> bus_selector3/1
  outpmodule/11(VOUTP_nEOPSpdReq_rpm) -> bus_creator/11
  bus_selector3/1 -> outpmodule/10(VEOP_bMotEnaReq_flg)  "<VEOP_bMotEnaReq_flg>"
  bus_selector3/2 -> outpmodule/11(VEOP_nEOPSpdReq_rpm)  "<VEOP_nEOPSpdReq_rpm>"
  BAPP_outputs/1 -> bus_selector1/1
  bus_selector2/2 -> outpmodule/9(VCRM_PwrEleAct_W)  "<VCRM_PwrEleAct_W>"
  BCRM_outputs/1 -> bus_selector2/1
  outpmodule/19(VOUTP_tqTMTqMin_Nm) -> bus_creator/19
  bus_selector1/6 -> outpmodule/6(VAPP_RotSpd_rpm)  "<VAPP_RotSpd_rpm>"
  bus_selector1/7 -> outpmodule/7(VAPP_OilTemp_degC)  "<VAPP_OilTemp_degC>"
  bus_selector2/1 -> outpmodule/8(VCRM_BusCurr_A)  "<VCRM_BusCurr_A>"
  bus_selector1/5 -> outpmodule/5(VAPP_uDC_V)  "<VAPP_uDC_V>"
  bus_selector1/2 -> outpmodule/2(VAPP_iQCurrAct_A)  "<VAPP_iQCurrAct_A>"
  bus_selector5/3 -> outpmodule/15(VOPM_MCUEna_flg)  "<VOPM_MCUEna_flg>"
  bus_selector1/3 -> outpmodule/3(VAPP_ADCKL30_V)  "<VAPP_ADCKL30_V>"
  bus_selector1/1 -> outpmodule/1(VAPP_iDCurrAct_A)  "<VAPP_iDCurrAct_A>"
  bus_selector5/1 -> outpmodule/13(VOPM_MotMod_enum)  "<VOPM_MotMod_enum>"
  outpmodule/9(VOUTP_PwrEleAct_W) -> bus_creator/9
  outpmodule/10(VOUTP_bMotEnaReq_flg) -> bus_creator/10
  outpmodule/7(VOUTP_OilTemp_degC) -> bus_creator/7
  outpmodule/6(VOUTP_RotSpd_rpm) -> bus_creator/6
  outpmodule/8(VOUTP_BusCurr_A) -> bus_creator/8
  outpmodule/4(VOUTP_ADCKL15_V) -> bus_creator/4
  outpmodule/5(VOUTP_uDC_V) -> bus_creator/5
  outpmodule/3(VOUTP_ADCKL30_V) -> bus_creator/3
  BLLC_outputs/1 -> bus_selector4/1
  outpmodule/2(VOUTP_iQCurrAct_A) -> bus_creator/2
  outpmodule/1(VOUTP_iDCurrAct_A) -> bus_creator/1
  BOPM_outputs/1 -> bus_selector5/1
  bus_selector6/2 -> outpmodule/19(VSYL_tqTMTqMin_Nm)  "<VSYL_tqTMTqMin_Nm>"
  BSYL_outputs/1 -> bus_selector6/1
  outpmodule/12(VOUTP_volfCooltFlowTar_C) -> bus_creator/12
  bus_selector6/1 -> outpmodule/18(VSYL_tqTMTqMax_Nm)  "<VSYL_tqTMTqMax_Nm>"
  bus_selector1/4 -> outpmodule/4(VAPP_ADCKL15_V)  "<VAPP_ADCKL15_V>"
  bus_selector5/5 -> outpmodule/17(VOPM_BoostOPSta_flg)  "<VOPM_BoostOPSta_flg>"

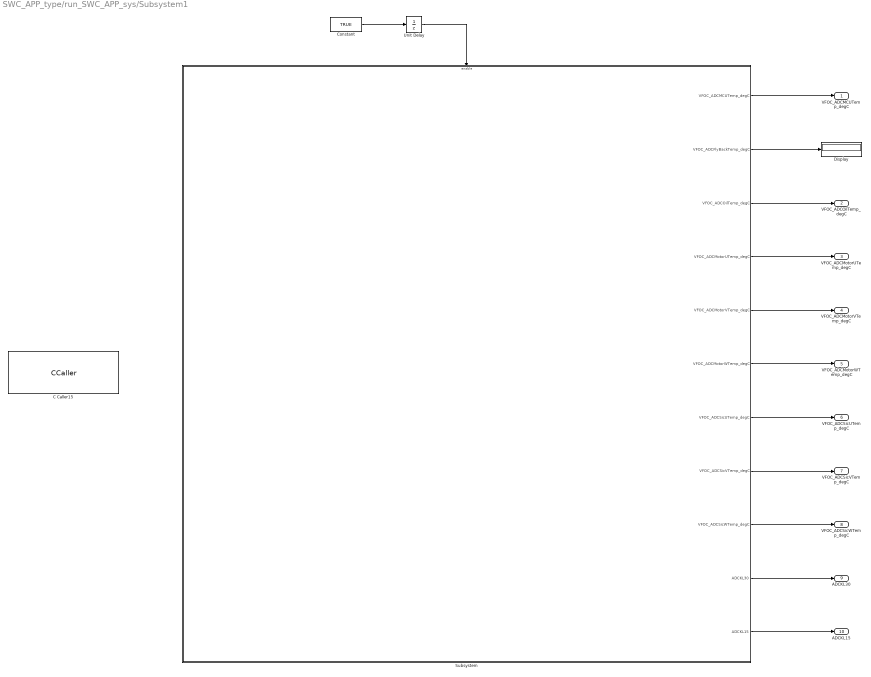
== system SWC_APP_type/run_SWC_APP_sys/Subsystem1 ==
  C Caller15 : CCaller  FunctionName=calculate_all_adc_system_signal
  Constant : Constant  Value=TRUE
  Display : Display
  Subsystem : Subsystem
  Unit Delay : UnitDelay  SampleTime=-1  HasFrameUpgradeWarning=on
  VFOC_ADCMCUTemp_degC : Outport
  VFOC_ADCOilTemp_degC : Outport  Port=2
  VFOC_ADCMotorUTemp_degC : Outport  Port=3
  VFOC_ADCMotorVTemp_degC : Outport  Port=4
  VFOC_ADCMotorWTemp_degC : Outport  Port=5
  VFOC_ADCSicUTemp_degC : Outport  Port=6
  VFOC_ADCSicVTemp_degC : Outport  Port=7
  VFOC_ADCSicWTemp_degC : Outport  Port=8
  ADCKL30 : Outport  Port=9
  ADCKL15 : Outport  Port=10
  wires:
  Constant/1 -> Unit Delay/1
  Unit Delay/1 -> Subsystem/Enable
  Subsystem/1(VFOC_ADCMCUTemp_degC) -> VFOC_ADCMCUTemp_degC/1
  Subsystem/2(VFOC_ADCFlyBackTemp_degC) -> Display/1
  Subsystem/3(VFOC_ADCOilTemp_degC) -> VFOC_ADCOilTemp_degC/1
  Subsystem/4(VFOC_ADCMotorUTemp_degC) -> VFOC_ADCMotorUTemp_degC/1
  Subsystem/5(VFOC_ADCMotorVTemp_degC) -> VFOC_ADCMotorVTemp_degC/1
  Subsystem/6(VFOC_ADCMotorWTemp_degC) -> VFOC_ADCMotorWTemp_degC/1
  Subsystem/7(VFOC_ADCSicUTemp_degC) -> VFOC_ADCSicUTemp_degC/1
  Subsystem/8(VFOC_ADCSicVTemp_degC) -> VFOC_ADCSicVTemp_degC/1
  Subsystem/9(VFOC_ADCSicWTemp_degC) -> VFOC_ADCSicWTemp_degC/1
  Subsystem/10(ADCKL30) -> ADCKL30/1
  Subsystem/11(ADCKL15) -> ADCKL15/1

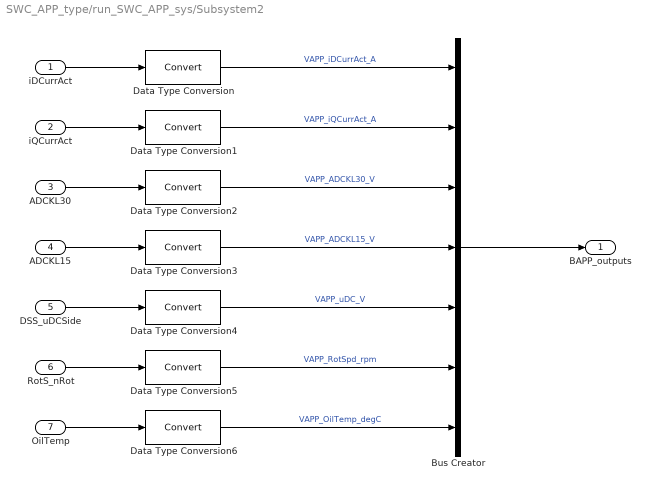
== system SWC_APP_type/run_SWC_APP_sys/Subsystem2 ==
  iDCurrAct : Inport
  iQCurrAct : Inport  Port=2
  ADCKL30 : Inport  Port=3
  ADCKL15 : Inport  Port=4
  DSS_uDCSide : Inport  Port=5
  RotS_nRot : Inport  Port=6
  OilTemp : Inport  Port=7
  Bus Creator : BusCreator  Inputs=7  OutDataTypeStr=Bus: BAPP_outputs  NonVirtualBus=on
  Data Type Conversion{,1..6} (7 alike) : DataTypeConversion  SaturateOnIntegerOverflow=off  RndMeth=Floor
  BAPP_outputs : Outport  OutDataTypeStr=Bus: BAPP_outputs
  wires:
  Data Type Conversion/1 -> Bus Creator/1  "VAPP_iDCurrAct_A"
  iQCurrAct/1 -> Data Type Conversion1/1
  iDCurrAct/1 -> Data Type Conversion/1
  Data Type Conversion1/1 -> Bus Creator/2  "VAPP_iQCurrAct_A"
  ADCKL30/1 -> Data Type Conversion2/1
  ADCKL15/1 -> Data Type Conversion3/1
  Data Type Conversion2/1 -> Bus Creator/3  "VAPP_ADCKL30_V"
  Data Type Conversion3/1 -> Bus Creator/4  "VAPP_ADCKL15_V"
  DSS_uDCSide/1 -> Data Type Conversion4/1
  Data Type Conversion4/1 -> Bus Creator/5  "VAPP_uDC_V"
  Data Type Conversion5/1 -> Bus Creator/6  "VAPP_RotSpd_rpm"
  Data Type Conversion6/1 -> Bus Creator/7  "VAPP_OilTemp_degC"
  RotS_nRot/1 -> Data Type Conversion5/1
  OilTemp/1 -> Data Type Conversion6/1
  Bus Creator/1 -> BAPP_outputs/1

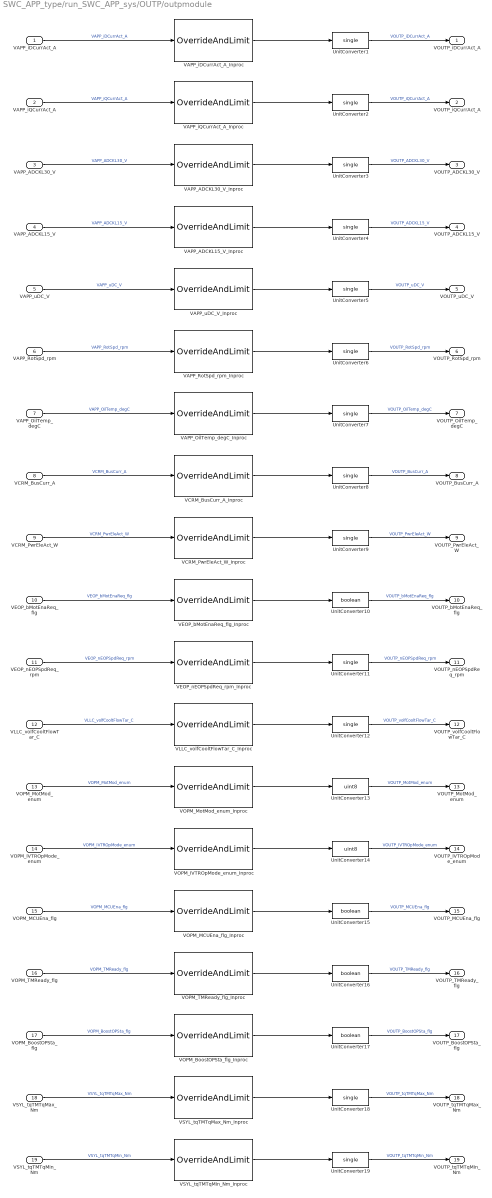
== system SWC_APP_type/run_SWC_APP_sys/OUTP/outpmodule ==
  VAPP_iDCurrAct_A : Inport
  VAPP_iQCurrAct_A : Inport  Port=2
  VAPP_ADCKL30_V : Inport  Port=3
  VAPP_ADCKL15_V : Inport  Port=4
  VAPP_uDC_V : Inport  Port=5
  VAPP_RotSpd_rpm : Inport  Port=6
  VAPP_OilTemp_degC : Inport  Port=7
  VCRM_BusCurr_A : Inport  Port=8
  VCRM_PwrEleAct_W : Inport  Port=9
  VEOP_bMotEnaReq_flg : Inport  Port=10
  VEOP_nEOPSpdReq_rpm : Inport  Port=11
  VLLC_volfCooltFlowTar_C : Inport  Port=12
  VOPM_MotMod_enum : Inport  Port=13
  VOPM_IVTROpMode_enum : Inport  Port=14
  VOPM_MCUEna_flg : Inport  Port=15
  VOPM_TMReady_flg : Inport  Port=16
  VOPM_BoostOPSta_flg : Inport  Port=17
  VSYL_tqTMTqMax_Nm : Inport  Port=18
  VSYL_tqTMTqMin_Nm : Inport  Port=19
  UnitConverter{1..9,11..12,18..19} (13 alike) : DataTypeConversion  OutDataTypeStr=single  SaturateOnIntegerOverflow=off  RndMeth=Floor
  UnitConverter{10,15..17} (4 alike) : DataTypeConversion  OutDataTypeStr=boolean  SaturateOnIntegerOverflow=off  RndMeth=Floor
  UnitConverter13 : DataTypeConversion  OutDataTypeStr=uint8  SaturateOnIntegerOverflow=off  RndMeth=Floor
  UnitConverter14 : DataTypeConversion  OutDataTypeStr=uint8  SaturateOnIntegerOverflow=off  RndMeth=Floor
  VAPP_ADCKL15_V_Inproc : FVT_lib/outp/OverrideAndLimit  SystemSampleTime=-1  VariantActivationTime=update diagram  AllowFlexibleInterface=on  Latency=0  AutoFrameSizeCalculation=off
      link override Signal_Limit/_maxval: Value=KOUTP_ADCKL15_V_maxval
      link override Signal_Limit/_minval: Value=KOUTP_ADCKL15_V_minval
      link override Signal_Override/_ovrdflg: Value=KOUTP_ADCKL15_V_ovrdflg
      link override Signal_Override/_ovrdval: Value=KOUTP_ADCKL15_V_ovrdval
  VAPP_ADCKL30_V_Inproc : FVT_lib/outp/OverrideAndLimit  SystemSampleTime=-1  VariantActivationTime=update diagram  AllowFlexibleInterface=on  Latency=0  AutoFrameSizeCalculation=off
      link override Signal_Limit/_maxval: Value=KOUTP_ADCKL30_V_maxval
      link override Signal_Limit/_minval: Value=KOUTP_ADCKL30_V_minval
      link override Signal_Override/_ovrdflg: Value=KOUTP_ADCKL30_V_ovrdflg
      link override Signal_Override/_ovrdval: Value=KOUTP_ADCKL30_V_ovrdval
  VAPP_OilTemp_degC_Inproc : FVT_lib/outp/OverrideAndLimit  SystemSampleTime=-1  VariantActivationTime=update diagram  AllowFlexibleInterface=on  Latency=0  AutoFrameSizeCalculation=off
      link override Signal_Limit/_maxval: Value=KOUTP_OilTemp_degC_maxval
      link override Signal_Limit/_minval: Value=KOUTP_OilTemp_degC_minval
      link override Signal_Override/_ovrdflg: Value=KOUTP_OilTemp_degC_ovrdflg
      link override Signal_Override/_ovrdval: Value=KOUTP_OilTemp_degC_ovrdval
  VAPP_RotSpd_rpm_Inproc : FVT_lib/outp/OverrideAndLimit  SystemSampleTime=-1  VariantActivationTime=update diagram  AllowFlexibleInterface=on  Latency=0  AutoFrameSizeCalculation=off
      link override Signal_Limit/_maxval: Value=KOUTP_RotSpd_rpm_maxval
      link override Signal_Limit/_minval: Value=KOUTP_RotSpd_rpm_minval
      link override Signal_Override/_ovrdflg: Value=KOUTP_RotSpd_rpm_ovrdflg
      link override Signal_Override/_ovrdval: Value=KOUTP_RotSpd_rpm_ovrdval
  VAPP_iDCurrAct_A_Inproc : FVT_lib/outp/OverrideAndLimit  SystemSampleTime=-1  VariantActivationTime=update diagram  AllowFlexibleInterface=on  Latency=0  AutoFrameSizeCalculation=off
      link override Signal_Limit/_maxval: Value=KOUTP_iDCurrAct_A_maxval
      link override Signal_Limit/_minval: Value=KOUTP_iDCurrAct_A_minval
      link override Signal_Override/_ovrdflg: Value=KOUTP_iDCurrAct_A_ovrdflg
      link override Signal_Override/_ovrdval: Value=KOUTP_iDCurrAct_A_ovrdval
  VAPP_iQCurrAct_A_Inproc : FVT_lib/outp/OverrideAndLimit  SystemSampleTime=-1  VariantActivationTime=update diagram  AllowFlexibleInterface=on  Latency=0  AutoFrameSizeCalculation=off
      link override Signal_Limit/_maxval: Value=KOUTP_iQCurrAct_A_maxval
      link override Signal_Limit/_minval: Value=KOUTP_iQCurrAct_A_minval
      link override Signal_Override/_ovrdflg: Value=KOUTP_iQCurrAct_A_ovrdflg
      link override Signal_Override/_ovrdval: Value=KOUTP_iQCurrAct_A_ovrdval
  VAPP_uDC_V_Inproc : FVT_lib/outp/OverrideAndLimit  SystemSampleTime=-1  VariantActivationTime=update diagram  AllowFlexibleInterface=on  Latency=0  AutoFrameSizeCalculation=off
      link override Signal_Limit/_maxval: Value=KOUTP_uDC_V_maxval
      link override Signal_Limit/_minval: Value=KOUTP_uDC_V_minval
      link override Signal_Override/_ovrdflg: Value=KOUTP_uDC_V_ovrdflg
      link override Signal_Override/_ovrdval: Value=KOUTP_uDC_V_ovrdval
  VCRM_BusCurr_A_Inproc : FVT_lib/outp/OverrideAndLimit  SystemSampleTime=-1  VariantActivationTime=update diagram  AllowFlexibleInterface=on  Latency=0  AutoFrameSizeCalculation=off
      link override Signal_Limit/_maxval: Value=KOUTP_BusCurr_A_maxval
      link override Signal_Limit/_minval: Value=KOUTP_BusCurr_A_minval
      link override Signal_Override/_ovrdflg: Value=KOUTP_BusCurr_A_ovrdflg
      link override Signal_Override/_ovrdval: Value=KOUTP_BusCurr_A_ovrdval
  VCRM_PwrEleAct_W_Inproc : FVT_lib/outp/OverrideAndLimit  SystemSampleTime=-1  VariantActivationTime=update diagram  AllowFlexibleInterface=on  Latency=0  AutoFrameSizeCalculation=off
      link override Signal_Limit/_maxval: Value=KOUTP_PwrEleAct_W_maxval
      link override Signal_Limit/_minval: Value=KOUTP_PwrEleAct_W_minval
      link override Signal_Override/_ovrdflg: Value=KOUTP_PwrEleAct_W_ovrdflg
      link override Signal_Override/_ovrdval: Value=KOUTP_PwrEleAct_W_ovrdval
  VEOP_bMotEnaReq_flg_Inproc : FVT_lib/outp/OverrideAndLimit  SystemSampleTime=-1  VariantActivationTime=update diagram  AllowFlexibleInterface=on  Latency=0  AutoFrameSizeCalculation=off
      link override Signal_Limit/_maxval: Value=KOUTP_bMotEnaReq_flg_maxval
      link override Signal_Limit/_minval: Value=KOUTP_bMotEnaReq_flg_minval
      link override Signal_Override/_ovrdflg: Value=KOUTP_bMotEnaReq_flg_ovrdflg
      link override Signal_Override/_ovrdval: Value=KOUTP_bMotEnaReq_flg_ovrdval
  VEOP_nEOPSpdReq_rpm_Inproc : FVT_lib/outp/OverrideAndLimit  SystemSampleTime=-1  VariantActivationTime=update diagram  AllowFlexibleInterface=on  Latency=0  AutoFrameSizeCalculation=off
      link override Signal_Limit/_maxval: Value=KOUTP_nEOPSpdReq_rpm_maxval
      link override Signal_Limit/_minval: Value=KOUTP_nEOPSpdReq_rpm_minval
      link override Signal_Override/_ovrdflg: Value=KOUTP_nEOPSpdReq_rpm_ovrdflg
      link override Signal_Override/_ovrdval: Value=KOUTP_nEOPSpdReq_rpm_ovrdval
  VLLC_volfCooltFlowTar_C_Inproc : FVT_lib/outp/OverrideAndLimit  SystemSampleTime=-1  VariantActivationTime=update diagram  AllowFlexibleInterface=on  Latency=0  AutoFrameSizeCalculation=off
      link override Signal_Limit/_maxval: Value=KOUTP_volfCooltFlowTar_C_maxval
      link override Signal_Limit/_minval: Value=KOUTP_volfCooltFlowTar_C_minval
      link override Signal_Override/_ovrdflg: Value=KOUTP_volfCooltFlowTar_C_ovrdflg
      link override Signal_Override/_ovrdval: Value=KOUTP_volfCooltFlowTar_C_ovrdval
  VOPM_BoostOPSta_flg_Inproc : FVT_lib/outp/OverrideAndLimit  SystemSampleTime=-1  VariantActivationTime=update diagram  AllowFlexibleInterface=on  Latency=0  AutoFrameSizeCalculation=off
      link override Signal_Limit/_maxval: Value=KOUTP_BoostOPSta_flg_maxval
      link override Signal_Limit/_minval: Value=KOUTP_BoostOPSta_flg_minval
      link override Signal_Override/_ovrdflg: Value=KOUTP_BoostOPSta_flg_ovrdflg
      link override Signal_Override/_ovrdval: Value=KOUTP_BoostOPSta_flg_ovrdval
  VOPM_IVTROpMode_enum_Inproc : FVT_lib/outp/OverrideAndLimit  SystemSampleTime=-1  VariantActivationTime=update diagram  AllowFlexibleInterface=on  Latency=0  AutoFrameSizeCalculation=off
      link override Signal_Limit/_maxval: Value=KOUTP_IVTROpMode_enum_maxval
      link override Signal_Limit/_minval: Value=KOUTP_IVTROpMode_enum_minval
      link override Signal_Override/_ovrdflg: Value=KOUTP_IVTROpMode_enum_ovrdflg
      link override Signal_Override/_ovrdval: Value=KOUTP_IVTROpMode_enum_ovrdval
  VOPM_MCUEna_flg_Inproc : FVT_lib/outp/OverrideAndLimit  SystemSampleTime=-1  VariantActivationTime=update diagram  AllowFlexibleInterface=on  Latency=0  AutoFrameSizeCalculation=off
      link override Signal_Limit/_maxval: Value=KOUTP_MCUEna_flg_maxval
      link override Signal_Limit/_minval: Value=KOUTP_MCUEna_flg_minval
      link override Signal_Override/_ovrdflg: Value=KOUTP_MCUEna_flg_ovrdflg
      link override Signal_Override/_ovrdval: Value=KOUTP_MCUEna_flg_ovrdval
  VOPM_MotMod_enum_Inproc : FVT_lib/outp/OverrideAndLimit  SystemSampleTime=-1  VariantActivationTime=update diagram  AllowFlexibleInterface=on  Latency=0  AutoFrameSizeCalculation=off
      link override Signal_Limit/_maxval: Value=KOUTP_MotMod_enum_maxval
      link override Signal_Limit/_minval: Value=KOUTP_MotMod_enum_minval
      link override Signal_Override/_ovrdflg: Value=KOUTP_MotMod_enum_ovrdflg
      link override Signal_Override/_ovrdval: Value=KOUTP_MotMod_enum_ovrdval
  VOPM_TMReady_flg_Inproc : FVT_lib/outp/OverrideAndLimit  SystemSampleTime=-1  VariantActivationTime=update diagram  AllowFlexibleInterface=on  Latency=0  AutoFrameSizeCalculation=off
      link override Signal_Limit/_maxval: Value=KOUTP_TMReady_flg_maxval
      link override Signal_Limit/_minval: Value=KOUTP_TMReady_flg_minval
      link override Signal_Override/_ovrdflg: Value=KOUTP_TMReady_flg_ovrdflg
      link override Signal_Override/_ovrdval: Value=KOUTP_TMReady_flg_ovrdval
  VSYL_tqTMTqMax_Nm_Inproc : FVT_lib/outp/OverrideAndLimit  SystemSampleTime=-1  VariantActivationTime=update diagram  AllowFlexibleInterface=on  Latency=0  AutoFrameSizeCalculation=off
      link override Signal_Limit/_maxval: Value=KOUTP_tqTMTqMax_Nm_maxval
      link override Signal_Limit/_minval: Value=KOUTP_tqTMTqMax_Nm_minval
      link override Signal_Override/_ovrdflg: Value=KOUTP_tqTMTqMax_Nm_ovrdflg
      link override Signal_Override/_ovrdval: Value=KOUTP_tqTMTqMax_Nm_ovrdval
  VSYL_tqTMTqMin_Nm_Inproc : FVT_lib/outp/OverrideAndLimit  SystemSampleTime=-1  VariantActivationTime=update diagram  AllowFlexibleInterface=on  Latency=0  AutoFrameSizeCalculation=off
      link override Signal_Limit/_maxval: Value=KOUTP_tqTMTqMin_Nm_maxval
      link override Signal_Limit/_minval: Value=KOUTP_tqTMTqMin_Nm_minval
      link override Signal_Override/_ovrdflg: Value=KOUTP_tqTMTqMin_Nm_ovrdflg
      link override Signal_Override/_ovrdval: Value=KOUTP_tqTMTqMin_Nm_ovrdval
  VOUTP_iDCurrAct_A : Outport
  VOUTP_iQCurrAct_A : Outport  Port=2
  VOUTP_ADCKL30_V : Outport  Port=3
  VOUTP_ADCKL15_V : Outport  Port=4
  VOUTP_uDC_V : Outport  Port=5
  VOUTP_RotSpd_rpm : Outport  Port=6
  VOUTP_OilTemp_degC : Outport  Port=7
  VOUTP_BusCurr_A : Outport  Port=8
  VOUTP_PwrEleAct_W : Outport  Port=9
  VOUTP_bMotEnaReq_flg : Outport  Port=10
  VOUTP_nEOPSpdReq_rpm : Outport  Port=11
  VOUTP_volfCooltFlowTar_C : Outport  Port=12
  VOUTP_MotMod_enum : Outport  Port=13
  VOUTP_IVTROpMode_enum : Outport  Port=14
  VOUTP_MCUEna_flg : Outport  Port=15
  VOUTP_TMReady_flg : Outport  Port=16
  VOUTP_BoostOPSta_flg : Outport  Port=17
  VOUTP_tqTMTqMax_Nm : Outport  Port=18
  VOUTP_tqTMTqMin_Nm : Outport  Port=19
  wires:
  VAPP_iDCurrAct_A/1 -> VAPP_iDCurrAct_A_Inproc/1  "VAPP_iDCurrAct_A"
  VAPP_iDCurrAct_A_Inproc/1 -> UnitConverter1/1
  UnitConverter1/1 -> VOUTP_iDCurrAct_A/1  "VOUTP_iDCurrAct_A"
  VAPP_iQCurrAct_A/1 -> VAPP_iQCurrAct_A_Inproc/1  "VAPP_iQCurrAct_A"
  VAPP_iQCurrAct_A_Inproc/1 -> UnitConverter2/1
  UnitConverter2/1 -> VOUTP_iQCurrAct_A/1  "VOUTP_iQCurrAct_A"
  VAPP_ADCKL30_V/1 -> VAPP_ADCKL30_V_Inproc/1  "VAPP_ADCKL30_V"
  VAPP_ADCKL30_V_Inproc/1 -> UnitConverter3/1
  UnitConverter3/1 -> VOUTP_ADCKL30_V/1  "VOUTP_ADCKL30_V"
  VAPP_ADCKL15_V/1 -> VAPP_ADCKL15_V_Inproc/1  "VAPP_ADCKL15_V"
  VAPP_ADCKL15_V_Inproc/1 -> UnitConverter4/1
  UnitConverter4/1 -> VOUTP_ADCKL15_V/1  "VOUTP_ADCKL15_V"
  VAPP_uDC_V/1 -> VAPP_uDC_V_Inproc/1  "VAPP_uDC_V"
  VAPP_uDC_V_Inproc/1 -> UnitConverter5/1
  UnitConverter5/1 -> VOUTP_uDC_V/1  "VOUTP_uDC_V"
  VAPP_RotSpd_rpm/1 -> VAPP_RotSpd_rpm_Inproc/1  "VAPP_RotSpd_rpm"
  VAPP_RotSpd_rpm_Inproc/1 -> UnitConverter6/1
  UnitConverter6/1 -> VOUTP_RotSpd_rpm/1  "VOUTP_RotSpd_rpm"
  VAPP_OilTemp_degC/1 -> VAPP_OilTemp_degC_Inproc/1  "VAPP_OilTemp_degC"
  VAPP_OilTemp_degC_Inproc/1 -> UnitConverter7/1
  UnitConverter7/1 -> VOUTP_OilTemp_degC/1  "VOUTP_OilTemp_degC"
  VCRM_BusCurr_A/1 -> VCRM_BusCurr_A_Inproc/1  "VCRM_BusCurr_A"
  VCRM_BusCurr_A_Inproc/1 -> UnitConverter8/1
  UnitConverter8/1 -> VOUTP_BusCurr_A/1  "VOUTP_BusCurr_A"
  VCRM_PwrEleAct_W/1 -> VCRM_PwrEleAct_W_Inproc/1  "VCRM_PwrEleAct_W"
  VCRM_PwrEleAct_W_Inproc/1 -> UnitConverter9/1
  UnitConverter9/1 -> VOUTP_PwrEleAct_W/1  "VOUTP_PwrEleAct_W"
  VEOP_bMotEnaReq_flg/1 -> VEOP_bMotEnaReq_flg_Inproc/1  "VEOP_bMotEnaReq_flg"
  VEOP_bMotEnaReq_flg_Inproc/1 -> UnitConverter10/1
  UnitConverter10/1 -> VOUTP_bMotEnaReq_flg/1  "VOUTP_bMotEnaReq_flg"
  VEOP_nEOPSpdReq_rpm/1 -> VEOP_nEOPSpdReq_rpm_Inproc/1  "VEOP_nEOPSpdReq_rpm"
  VEOP_nEOPSpdReq_rpm_Inproc/1 -> UnitConverter11/1
  UnitConverter11/1 -> VOUTP_nEOPSpdReq_rpm/1  "VOUTP_nEOPSpdReq_rpm"
  VLLC_volfCooltFlowTar_C/1 -> VLLC_volfCooltFlowTar_C_Inproc/1  "VLLC_volfCooltFlowTar_C"
  VLLC_volfCooltFlowTar_C_Inproc/1 -> UnitConverter12/1
  UnitConverter12/1 -> VOUTP_volfCooltFlowTar_C/1  "VOUTP_volfCooltFlowTar_C"
  VOPM_MotMod_enum/1 -> VOPM_MotMod_enum_Inproc/1  "VOPM_MotMod_enum"
  VOPM_MotMod_enum_Inproc/1 -> UnitConverter13/1
  UnitConverter13/1 -> VOUTP_MotMod_enum/1  "VOUTP_MotMod_enum"
  VOPM_IVTROpMode_enum/1 -> VOPM_IVTROpMode_enum_Inproc/1  "VOPM_IVTROpMode_enum"
  VOPM_IVTROpMode_enum_Inproc/1 -> UnitConverter14/1
  UnitConverter14/1 -> VOUTP_IVTROpMode_enum/1  "VOUTP_IVTROpMode_enum"
  VOPM_MCUEna_flg/1 -> VOPM_MCUEna_flg_Inproc/1  "VOPM_MCUEna_flg"
  VOPM_MCUEna_flg_Inproc/1 -> UnitConverter15/1
  UnitConverter15/1 -> VOUTP_MCUEna_flg/1  "VOUTP_MCUEna_flg"
  VOPM_TMReady_flg/1 -> VOPM_TMReady_flg_Inproc/1  "VOPM_TMReady_flg"
  VOPM_TMReady_flg_Inproc/1 -> UnitConverter16/1
  UnitConverter16/1 -> VOUTP_TMReady_flg/1  "VOUTP_TMReady_flg"
  VOPM_BoostOPSta_flg/1 -> VOPM_BoostOPSta_flg_Inproc/1  "VOPM_BoostOPSta_flg"
  VOPM_BoostOPSta_flg_Inproc/1 -> UnitConverter17/1
  UnitConverter17/1 -> VOUTP_BoostOPSta_flg/1  "VOUTP_BoostOPSta_flg"
  VSYL_tqTMTqMax_Nm/1 -> VSYL_tqTMTqMax_Nm_Inproc/1  "VSYL_tqTMTqMax_Nm"
  VSYL_tqTMTqMax_Nm_Inproc/1 -> UnitConverter18/1
  UnitConverter18/1 -> VOUTP_tqTMTqMax_Nm/1  "VOUTP_tqTMTqMax_Nm"
  VSYL_tqTMTqMin_Nm/1 -> VSYL_tqTMTqMin_Nm_Inproc/1  "VSYL_tqTMTqMin_Nm"
  VSYL_tqTMTqMin_Nm_Inproc/1 -> UnitConverter19/1
  UnitConverter19/1 -> VOUTP_tqTMTqMin_Nm/1  "VOUTP_tqTMTqMin_Nm"
